simulink model "RoadTestingVelocityandThreat_RRT"  (Simulink 8.0)
settings: Solver=ode3  StartTime=0.0  StopTime=30  FixedStep=.05  RelTol=1e-3
StartFcn:
  | Threshold = 11;
  | MaxCluster = 25;
  | Num_Beams = 726;
  | Road_Width = 10;
  | Cone_Area = 0.125;
  | Cone_Spacing = 4;
  | Scaling = 1.1;
  | areaBuffer = 0.05;
  | spacingBuffer = 0.05;
  | RoadfromConeoffset = 0.5;
  | threatThreshold = 75;
  | distThreshold = 5;
  | minSpeed = 2.0;
  | minDistance = 1.0;
  | threatConeAngle = 70;
  | allowableDistToCone = 1.5;
  | thresholdManueverAngle = 27.5;
  | maxStepSize = 0.65;
  | aspectRatioBuffer =2;
  | javaaddpath({'/'});
  | import ClusterMethodWithVelocityThreat.*;
  | DataCluster = ClusterMethodWithVelocityThreat(Threshold,MaxCluster,Scaling,...
  | Road_Width,Cone_Area,Cone_Spacing,areaBuffer,spacingBuffer,RoadfromConeoffset,threatThreshold,...
  | distThreshold,minSpeed,minDistance,threatConeAngle,allowableDistToCone,thresholdManueverAngle,maxStepSize,aspectRatioBuffer);
  | %DataCluster = ClusterMethodWithVelocityThreatWorking(Threshold,MaxCluster,Scaling,...
  | %Road_Width,Cone_Area,Cone_Spacing,areaBuffer,spacingBuffer,RoadfromConeoffset,threatThreshold,...
  | %distThreshold,minSpeed,minDistance,threatConeAngle,allowableDistToCone);
  | eml.extrinsic('evalin');
StopFcn:
  | clear DataCluster;
  | clear Threshold;
  | clear MaxCluster;
  | clear Num_Beams;
  | clear Road_Width;
  | clear Cone_Area;
  | clear Cone_Spacing;
  | clear Scaling;
  | clear areaBuffer;
  | clear spacingBuffer;
  | clear RoadfromConeoffset;
  | clear threatThreshold;
  | clear distThreshold;
  | clear minSpeed;
  | clear minDistance;
  | clear threatConeAngle;
  | clear allowableDistToCone;
  | clear thresholdManueverAngle;
  | clear maxStepSize;
  | clear aspectRatioBuffer;
settings Model: Creator=Thomas  LastModifiedBy=Thomas
settings DataIOCC: SignalLoggingSaveFormat=ModelDataLogs
settings DebuggingCC: FcnCallInpInsideContextMsg=EnableAllAsWarning
settings GRTTargetCC: CombineOutputUpdateFcns=off  GRTInterface=on

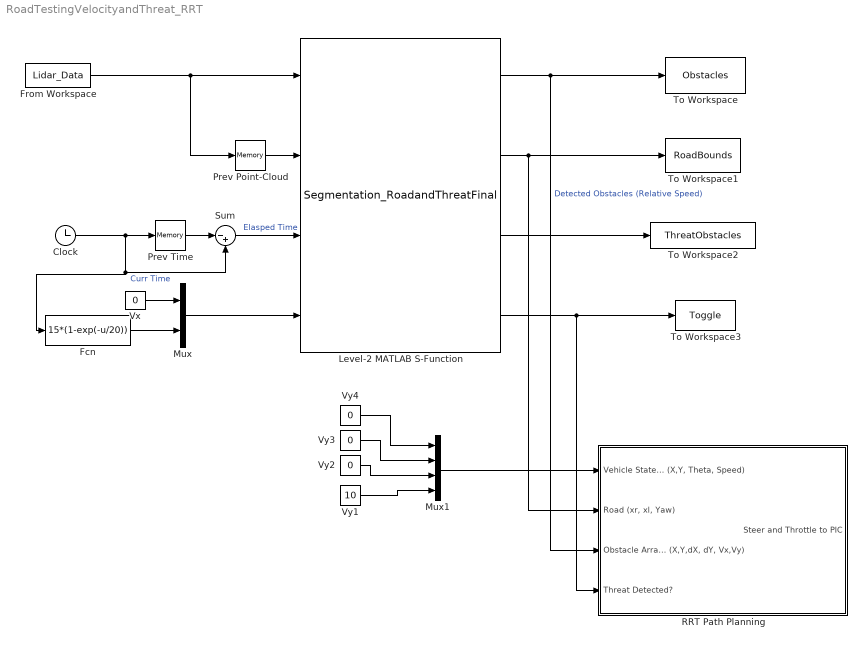
== system RoadTestingVelocityandThreat_RRT ==
  Clock : Clock
  Fcn : Fcn  Expr=15*(1-exp(-u/20))
  From Workspace : FromWorkspace  VariableName=Lidar_Data  SampleTime=0  OutputAfterFinalValue=Setting to zero
  Level-2 MATLAB S-Function : M-S-Function  FunctionName=Segmentation_RoadandThreatFinal
  Mux : Mux  Inputs=2
  Mux1 : Mux
  Prev Point-Cloud : Memory
  Prev Time : Memory
  RRT Path Planning : Subsystem
  Sum : Sum  Inputs=|-+
  To Workspace : ToWorkspace  VariableName=Obstacles  SampleTime=-1  SaveFormat=Structure With Time
  To Workspace1 : ToWorkspace  VariableName=RoadBounds  SampleTime=-1  SaveFormat=Structure With Time
  To Workspace2 : ToWorkspace  VariableName=ThreatObstacles  SampleTime=-1  SaveFormat=Structure With Time
  To Workspace3 : ToWorkspace  VariableName=Toggle  SampleTime=-1  SaveFormat=Structure With Time
  Vx : Constant  Value=0
  Vy1 : Constant  Value=10
  Vy2 : Constant  Value=0
  Vy3 : Constant  Value=0
  Vy4 : Constant  Value=0
  wires:
  Prev Time/1 -> Sum/1
  Sum/1 -> Level-2 MATLAB S-Function/3  "Elasped Time"
  Clock/1 -> Prev Time/1, Fcn/1, Sum/2  "Curr Time"
  Prev Point-Cloud/1 -> Level-2 MATLAB S-Function/2
  Level-2 MATLAB S-Function/1 -> RRT Path Planning/3("Obstacle Array (X,Y,dX, dY, Vx,Vy)"), To Workspace/1  "Detected Obstacles (Relative Speed)"
  Level-2 MATLAB S-Function/2 -> RRT Path Planning/2("Road (xr, xl, Yaw)"), To Workspace1/1
  Vx/1 -> Mux/1
  Fcn/1 -> Mux/2
  From Workspace/1 -> Prev Point-Cloud/1, Level-2 MATLAB S-Function/1
  Mux/1 -> Level-2 MATLAB S-Function/4
  Level-2 MATLAB S-Function/3 -> To Workspace2/1
  Level-2 MATLAB S-Function/4 -> RRT Path Planning/4(Threat Detected?), To Workspace3/1
  Mux1/1 -> RRT Path Planning/1("Vehicle State (X,Y, Theta, Speed)")
  Vy1/1 -> Mux1/4
  Vy4/1 -> Mux1/1
  Vy3/1 -> Mux1/2
  Vy2/1 -> Mux1/3

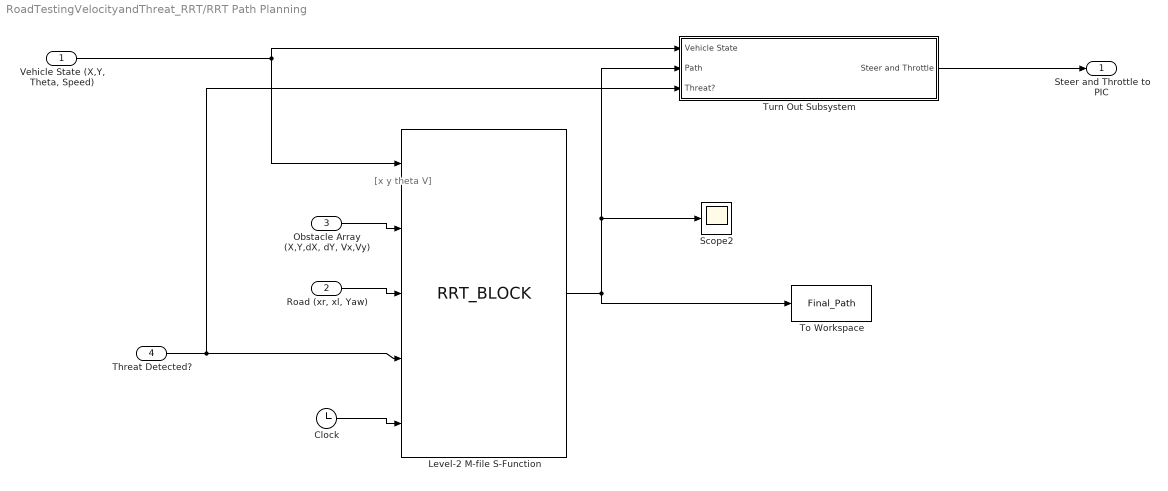
== system RoadTestingVelocityandThreat_RRT/RRT Path Planning ==
  note: [x y theta V]
  "Vehicle State (X,Y, Theta, Speed)" : Inport
  "Road (xr, xl, Yaw)" : Inport  Port=2
  "Obstacle Array (X,Y,dX, dY, Vx,Vy)" : Inport  Port=3
  Threat Detected? : Inport  Port=4
  Clock : Clock
  Level-2 M-file S-Function : M-S-Function  FunctionName=RRT_BLOCK  Parameters=6
  Scope2 : Scope
      settings: SaveName=ScopeData5
  To Workspace : ToWorkspace  VariableName=Final_Path  SampleTime=-1  SaveFormat=Structure With Time
  Turn Out Subsystem : Subsystem
  Steer and Throttle to PIC : Outport
  wires:
  Clock/1 -> Level-2 M-file S-Function/5
  "Vehicle State (X,Y, Theta, Speed)"/1 -> Level-2 M-file S-Function/1, Turn Out Subsystem/1(Vehicle State)
  "Obstacle Array (X,Y,dX, dY, Vx,Vy)"/1 -> Level-2 M-file S-Function/2
  Turn Out Subsystem/1(Steer and Throttle) -> Steer and Throttle to PIC/1
  Threat Detected?/1 -> Level-2 M-file S-Function/4, Turn Out Subsystem/3(Threat?)
  "Road (xr, xl, Yaw)"/1 -> Level-2 M-file S-Function/3
  Level-2 M-file S-Function/1 -> Turn Out Subsystem/2(Path), Scope2/1, To Workspace/1

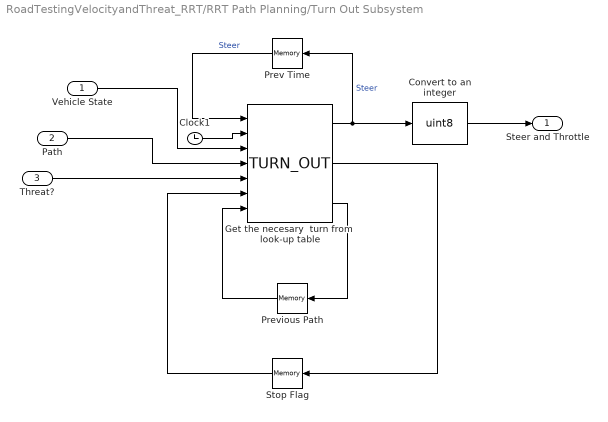
== system RoadTestingVelocityandThreat_RRT/RRT Path Planning/Turn Out Subsystem ==
  Vehicle State : Inport
  Path : Inport  Port=2
  Threat? : Inport  Port=3
  Clock1 : Clock
  Convert to an integer : DataTypeConversion  OutDataTypeStr=uint8  SampleTime=.05  SaturateOnIntegerOverflow=on  RndMeth=Zero
  Get the necesary  turn from  look-up table : M-S-Function  FunctionName=TURN_OUT  Parameters=4
  Prev Time : Memory  X0=[250 0 0]
  Previous Path : Memory  X0=zeros(50,5)
  Stop Flag : Memory
  Steer and Throttle : Outport
  wires:
  Get the necesary  turn from  look-up table/1 -> Prev Time/1, Convert to an integer/1  "Steer"
  Convert to an integer/1 -> Steer and Throttle/1
  Prev Time/1 -> Get the necesary  turn from  look-up table/1  "Steer"
  Get the necesary  turn from  look-up table/2 -> Stop Flag/1
  Clock1/1 -> Get the necesary  turn from  look-up table/2
  Stop Flag/1 -> Get the necesary  turn from  look-up table/6
  Vehicle State/1 -> Get the necesary  turn from  look-up table/3
  Get the necesary  turn from  look-up table/3 -> Previous Path/1
  Previous Path/1 -> Get the necesary  turn from  look-up table/7
  Path/1 -> Get the necesary  turn from  look-up table/4
  Threat?/1 -> Get the necesary  turn from  look-up table/5
